simulink model "addFM"  (R2026a)
settings: configuration reference "standardSILConfiguraitonParams" (kept outside this file)
undefined symbols (not defined in the file or in its folder): aircraftInitialEuler_rad
libraries: simulink x2
settings Model: Creator=GTAR  LastModifiedBy=Edison Altamirano
settings ConfigSetRef: SourceName=standardSILConfiguraitonParams  SourceLocation=Base Workspace

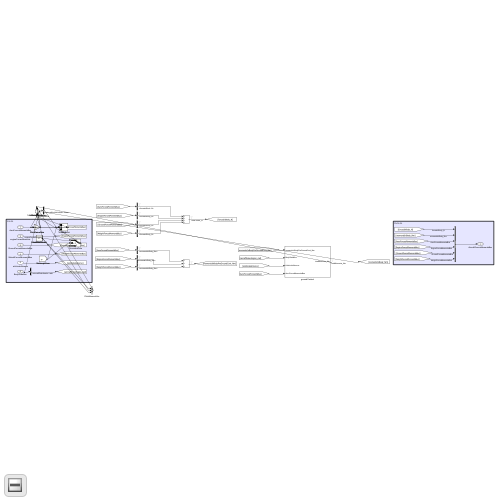
[thumbnail: Simulink's stored preview of the top-level diagram]
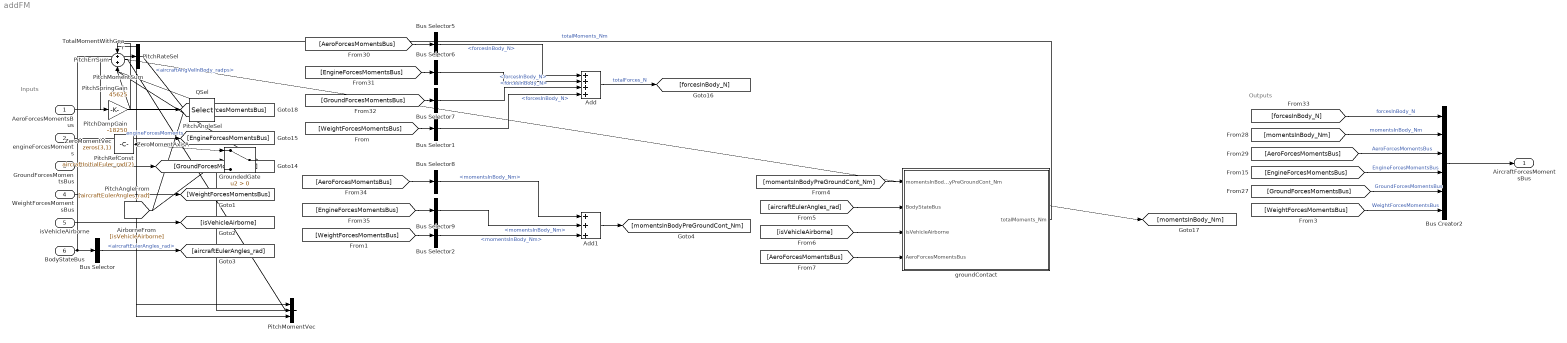
== system addFM ==
  note: Inputs
  note: Outputs
  AeroForcesMomentsBus : Inport  OutDataTypeStr=Bus: ComponentForcesMomentsBus  SampleTime=0
  engineForcesMoments : Inport  Port=2  OutDataTypeStr=Bus: ComponentForcesMomentsBus
  GroundForcesMomentsBus : Inport  Port=3  OutDataTypeStr=Bus: ComponentForcesMomentsBus  SampleTime=0
  WeightForcesMomentsBus : Inport  Port=4  OutDataTypeStr=Bus: ComponentForcesMomentsBus  SampleTime=0
  isVehicleAirborne : Inport  Port=5  OutDataTypeStr=boolean
  BodyStateBus : Inport  Port=6  OutDataTypeStr=Bus: BodyStateBus  SampleTime=0  BusOutputAsStruct=on
  Add : Sum  Inputs=++++
  Add1 : Sum  Inputs=+++
  Bus Creator2 : BusCreator  Inputs=6  OutDataTypeStr=Bus: AircraftForcesMomentsBus
  Bus Selector : BusSelector  OutputSignals=aircraftEulerAngles_rad
  Bus Selector{1,5..7} (4 alike) : BusSelector  OutputSignals=forcesInBody_N
  Bus Selector2 : BusSelector  OutputSignals=momentsInBody_Nm
  Bus Selector8 : BusSelector  OutputSignals=momentsInBody_Nm
  Bus Selector9 : BusSelector  OutputSignals=momentsInBody_Nm
  GroundedGate : Switch  Criteria=u2 > Threshold  SaturateOnIntegerOverflow=off  InputSameDT=off
  PitchAngleSel : Selector  InputPortWidth=3  IndexOptions=Index vector (dialog)  Indices=[2]  OutputSizes=1
  PitchDampGain : Gain  Gain=-18250
  PitchErrSum : Sum  Inputs=+-
  PitchMomentSum : Sum
  PitchMomentVec : Concatenate  NumInputs=3
  PitchRateSel : BusSelector  OutputSignals=aircraftAngVelInBody_radps
  PitchRefConst : Constant  Value=aircraftInitialEuler_rad(2)
  PitchSpringGain : Gain  Gain=45625
  QSel : Selector  InputPortWidth=3  IndexOptions=Index vector (dialog)  Indices=[2]  OutputSizes=1
  TotalMomentWithGear : Sum
  ZeroMomentAxisA : Constant  Value=0
  ZeroMomentVec : Constant  Value=zeros(3,1)
  groundContact : Subsystem
  AircraftForcesMomentsBus : Outport  OutDataTypeStr=Bus: AircraftForcesMomentsBus  SampleTime=0
  wires:
  [forcesInBody_N] -> Bus Creator2/1  "forcesInBody_N"
  Bus Selector6/1 -> Add/2  "<forcesInBody_N>"
  [EngineForcesMomentsBus] -> Bus Creator2/4  "EngineForcesMomentsBus"
  [EngineForcesMomentsBus] -> Bus Selector9/1
  Bus Selector7/1 -> Add/3  "<forcesInBody_N>"
  [AeroForcesMomentsBus] -> Bus Selector5/1
  Bus Selector9/1 -> Add1/2  "<momentsInBody_Nm>"
  Add/1 -> [forcesInBody_N]  "totalForces_N"
  [AeroForcesMomentsBus] -> Bus Creator2/3  "AeroForcesMomentsBus"
  Bus Selector8/1 -> Add1/1  "<momentsInBody_Nm>"
  [momentsInBody_Nm] -> Bus Creator2/2  "momentsInBody_Nm"
  Bus Creator2/1 -> AircraftForcesMomentsBus/1
  [GroundForcesMomentsBus] -> Bus Selector7/1
  engineForcesMoments/1 -> [EngineForcesMomentsBus]  "engineForcesMoments"
  [AeroForcesMomentsBus] -> Bus Selector8/1
  [EngineForcesMomentsBus] -> Bus Selector6/1
  [GroundForcesMomentsBus] -> Bus Creator2/5  "GroundForcesMomentsBus"
  AeroForcesMomentsBus/1 -> [AeroForcesMomentsBus]
  GroundForcesMomentsBus/1 -> [GroundForcesMomentsBus]
  WeightForcesMomentsBus/1 -> [WeightForcesMomentsBus]
  [WeightForcesMomentsBus] -> Bus Selector1/1
  Bus Selector1/1 -> Add/4  "<forcesInBody_N>"
  [WeightForcesMomentsBus] -> Bus Selector2/1
  Bus Selector2/1 -> Add1/3  "<momentsInBody_Nm>"
  [WeightForcesMomentsBus] -> Bus Creator2/6  "WeightForcesMomentsBus"
  Bus Selector5/1 -> Add/1  "<forcesInBody_N>"
  isVehicleAirborne/1 -> [isVehicleAirborne]
  Add1/1 -> [momentsInBodyPreGroundCont_Nm]
  BodyStateBus/1 -> Bus Selector/1, PitchRateSel/1
  Bus Selector/1 -> [aircraftEulerAngles_rad]  "<aircraftEulerAngles_rad>"
  [momentsInBodyPreGroundCont_Nm] -> groundContact/1(momentsInBodyPreGroundCont_Nm)
  [aircraftEulerAngles_rad] -> groundContact/2(BodyStateBus)
  [isVehicleAirborne] -> groundContact/3(isVehicleAirborne)
  [AeroForcesMomentsBus] -> groundContact/4(AeroForcesMomentsBus)
  [aircraftEulerAngles_rad] -> PitchAngleSel/1
  PitchRateSel/1 -> QSel/1  "<aircraftAngVelInBody_radps>"
  PitchRefConst/1 -> PitchErrSum/1
  PitchAngleSel/1 -> PitchErrSum/2
  PitchErrSum/1 -> PitchSpringGain/1
  QSel/1 -> PitchDampGain/1
  PitchSpringGain/1 -> PitchMomentSum/1
  PitchDampGain/1 -> PitchMomentSum/2
  ZeroMomentAxisA/1 -> PitchMomentVec/1, PitchMomentVec/3
  PitchMomentSum/1 -> PitchMomentVec/2
  ZeroMomentVec/1 -> GroundedGate/1
  [isVehicleAirborne] -> GroundedGate/2
  PitchMomentVec/1 -> GroundedGate/3
  groundContact/1(totalMoments_Nm) -> TotalMomentWithGear/1  "totalMoments_Nm"
  GroundedGate/1 -> TotalMomentWithGear/2
  TotalMomentWithGear/1 -> [momentsInBody_Nm]

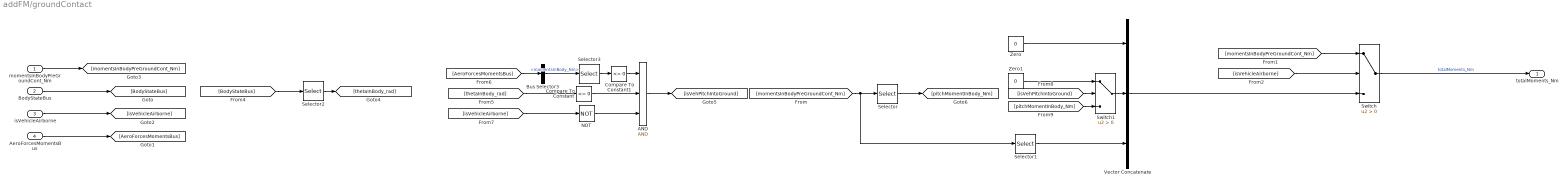
== system addFM/groundContact ==
  momentsInBodyPreGroundCont_Nm : Inport
  BodyStateBus : Inport  Port=2
  isVehicleAirborne : Inport  Port=3
  AeroForcesMomentsBus : Inport  Port=4
  AND : Logic  Inputs=3  AllPortsSameDT=off  OutDataTypeStr=boolean
  Bus Selector3 : BusSelector  OutputSignals=momentsInBody_Nm
  Compare To Constant : simulink/Logic and Bit Operations/Compare To Constant  relop=<=  const=0  OutDataTypeStr=boolean
  Compare To Constant1 : simulink/Logic and Bit Operations/Compare To Constant  relop=<=  const=0  OutDataTypeStr=boolean
  NOT : Logic  Operator=NOT  IconShape=distinctive  AllPortsSameDT=off  OutDataTypeStr=boolean
  Selector : Selector  InputPortWidth=3  IndexOptions=Index vector (dialog)  Indices=2  OutputSizes=1
  Selector1 : Selector  InputPortWidth=3  IndexOptions=Index vector (dialog)  Indices=3  OutputSizes=1
  Selector2 : Selector  InputPortWidth=3  IndexOptions=Index vector (dialog)  Indices=2  OutputSizes=1
  Selector3 : Selector  InputPortWidth=3  IndexOptions=Index vector (dialog)  Indices=2  OutputSizes=1
  Switch : Switch  Criteria=u2 > Threshold  SaturateOnIntegerOverflow=off  InputSameDT=off
  Switch1 : Switch  Criteria=u2 > Threshold  SaturateOnIntegerOverflow=off  InputSameDT=off
  Vector Concatenate : Concatenate  NumInputs=3
  Zero : Constant  Value=0  OutDataTypeStr=Inherit: Inherit via back propagation
  Zero1 : Constant  Value=0  OutDataTypeStr=Inherit: Inherit via back propagation
  totalMoments_Nm : Outport
  wires:
  NOT/1 -> AND/3
  [BodyStateBus] -> Selector2/1
  Compare To Constant/1 -> AND/2
  [thetaInBody_rad] -> Compare To Constant/1
  [isVehicleAirborne] -> NOT/1
  Compare To Constant1/1 -> AND/1
  AND/1 -> [isVehPitchIntoGround]
  [AeroForcesMomentsBus] -> Bus Selector3/1
  Selector3/1 -> Compare To Constant1/1
  Bus Selector3/1 -> Selector3/1  "<momentsInBody_Nm>"
  Selector2/1 -> [thetaInBody_rad]
  [isVehPitchIntoGround] -> Switch1/2
  Zero/1 -> Vector Concatenate/1
  [momentsInBodyPreGroundCont_Nm] -> Selector/1, Selector1/1
  Selector/1 -> [pitchMomentInBody_Nm]
  Switch1/1 -> Vector Concatenate/2
  Selector1/1 -> Vector Concatenate/3
  Zero1/1 -> Switch1/1
  [pitchMomentInBody_Nm] -> Switch1/3
  BodyStateBus/1 -> [BodyStateBus]
  AeroForcesMomentsBus/1 -> [AeroForcesMomentsBus]
  isVehicleAirborne/1 -> [isVehicleAirborne]
  momentsInBodyPreGroundCont_Nm/1 -> [momentsInBodyPreGroundCont_Nm]
  [isVehicleAirborne] -> Switch/2
  Vector Concatenate/1 -> Switch/3
  Switch/1 -> totalMoments_Nm/1  "totalMoments_Nm"
  [momentsInBodyPreGroundCont_Nm] -> Switch/1
